simulink model "webcamT"  (R2019a)
settings: Solver=VariableStepAuto  StartTime=0.0  StopTime=inf  RelTol=1e-3
undefined symbols (not defined in the file or in its folder): none, Rec, SDTV, videoinput
libraries: visionconversions x1, imaqlib x1, visionanalysis x1, simulink x1
settings Model: Creator=Pola  LastModifiedBy=Pola

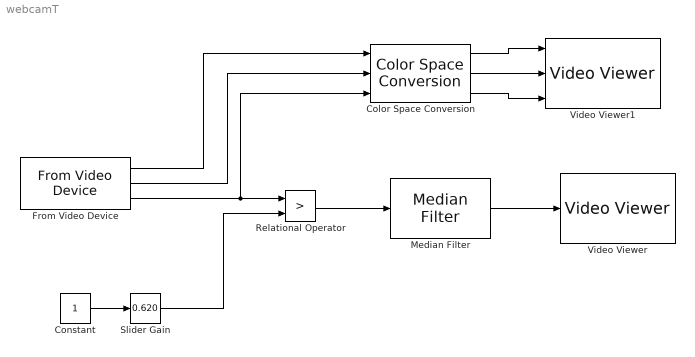
== system webcamT ==
  Color Space Conversion : visionconversions/Color Space  Conversion  conversion=Obsolete  conversionActive=Y'CbCr to R'G'B'  wp_str=D65  rec=Rec. 601 (SDTV)  sys=1125/60/2:1  imagePorts=Separate color signals
  Constant : Constant
  From Video Device : imaqlib/From Video Device  DeviceMenu=winvideo 2 (USB Camera)  Device=winvideo 2 (USB Camera)  ObjConstructor=videoinput('winvideo', 2)  VideoFormatMenu=YUY2_1024x576  VideoFormat=YUY2_1024x576  VideoSource=input1  ROIPosition=[0 0 576 1024]  EnableHWTrigger=off  TriggerConfiguration=none/none  SampleTime=1/30  OutputPortsMode=Separate color signals  DataType=single  CanDoHWTrigger=no  ReturnedColorSpace=YCbCr  BlockHandle=25.0002  ROIWidth=1024  ROIHeight=576  ROIColumn=0  ROIRow=0  EngXMLPath=D:\matlab2019\toolbox\imaq\imaq\private  DevXMLPath=C:\ProgramData\MATLAB\SupportPackages\R2019a\toolbox\imaq\supportpackages\genericvideo\adaptor\win64  EngLibPath=D:\matlab2019\toolbox\imaq\imaqblks\imaqmex\win64  ColorSpace=YCbCr  BayerSensorAlignment=grbg  ImaqMode=on
      settings: SourceProductName=Image Acquisition Toolbox
  Median Filter : visionanalysis/Median Filter  nghbood=[3 3]  outSize=Same as input port I  padType=Constant  padSrc=Specify via dialog  padVal=0  roundingMode=Floor  overflowMode=off  prodOutputSlope=2^-30  accumSlope=2^-30  outputSlope=2^-15
      settings: SourceProductName=Computer Vision Toolbox  SourceProductBaseCode=VP
  Relational Operator : RelationalOperator  Operator=>  OutDataTypeStr=boolean  RndMeth=Simplest
  Slider Gain : simulink/Math Operations/Slider Gain  gain=0.620  low=0  high=2
  Video Viewer : VideoViewer  FigPos=[1031.4 574.8 417.6 304]
  Video Viewer1 : VideoViewer  imagePorts=separate color signals  FigPos=[599.4 574.8 417.6 304]
  wires:
  From Video Device/3 -> Color Space Conversion/3, Relational Operator/1
  Constant/1 -> Slider Gain/1
  Slider Gain/1 -> Relational Operator/2
  From Video Device/1 -> Color Space Conversion/1
  From Video Device/2 -> Color Space Conversion/2
  Color Space Conversion/1 -> Video Viewer1/1
  Color Space Conversion/2 -> Video Viewer1/2
  Color Space Conversion/3 -> Video Viewer1/3
  Relational Operator/1 -> Median Filter/1
  Median Filter/1 -> Video Viewer/1
